simulink model "models"  (R2024a)
settings: Solver=VariableStepAuto  StartTime=0.0  StopTime=10.0  RelTol=1e-3
undefined symbols (not defined in the file): ic
libraries: cstblocks x2
settings Model: Creator=tinnovosel  LastModifiedBy=tinnovosel

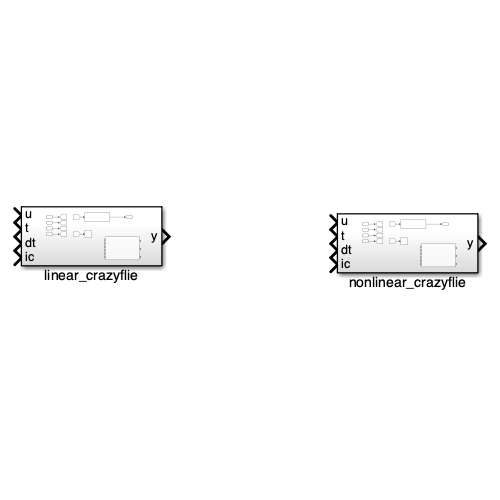
[thumbnail: Simulink's stored preview of the top-level diagram]
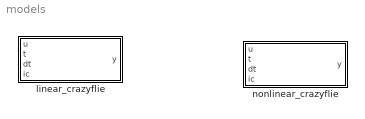
== system models ==
  linear_crazyflie : Subsystem
  nonlinear_crazyflie : Subsystem

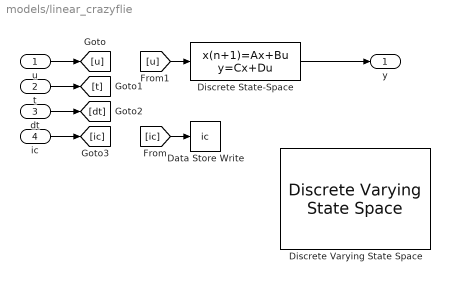
== system models/linear_crazyflie ==
  u : Inport
  t : Inport  Port=2
  dt : Inport  Port=3
  ic : Inport  Port=4
  Data Store Write : DataStoreWrite  DataStoreName=ic  IndexOptions=Index vector (dialog)  Indices=1  OutputSizes=1
  Discrete State-Space : DiscreteStateSpace  InitialCondition=ic  SampleTime=-1
  Discrete Varying State Space : cstblocks/Linear Parameter Varying/Discrete Varying State Space  x0=0  Ts=-1  OutputX=on  OutputDX=on  Feedthrough=on  InputX0=on  InputDX0=off  InputU0=off  InputY0=off
  y : Outport
  wires:
  u/1 -> [u]
  t/1 -> [t]
  dt/1 -> [dt]
  ic/1 -> [ic]
  [ic] -> Data Store Write/1
  [u] -> Discrete State-Space/1
  Discrete State-Space/1 -> y/1

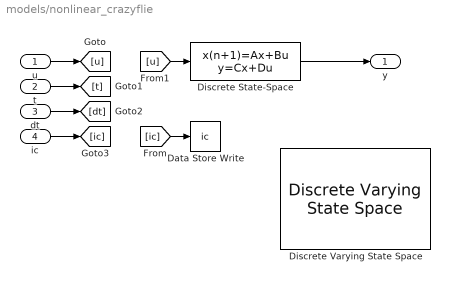
== system models/nonlinear_crazyflie ==
  u : Inport
  t : Inport  Port=2
  dt : Inport  Port=3
  ic : Inport  Port=4
  Data Store Write : DataStoreWrite  DataStoreName=ic  IndexOptions=Index vector (dialog)  Indices=1  OutputSizes=1
  Discrete State-Space : DiscreteStateSpace  InitialCondition=ic  SampleTime=-1
  Discrete Varying State Space : cstblocks/Linear Parameter Varying/Discrete Varying State Space  x0=0  Ts=-1  OutputX=on  OutputDX=on  Feedthrough=on  InputX0=on  InputDX0=off  InputU0=off  InputY0=off
  y : Outport
  wires:
  Discrete State-Space/1 -> y/1
  [u] -> Discrete State-Space/1
  [ic] -> Data Store Write/1
  ic/1 -> [ic]
  dt/1 -> [dt]
  t/1 -> [t]
  u/1 -> [u]
